simulink model "untitled0"  (R2023a)
settings: Solver=FixedStepAuto  StartTime=0.0  StopTime=3  FixedStep=1e-5  RelTol=1e-3
undefined symbols (not defined in the file): J, Ki, Kiv, Kp, Kpv, KT, La, Ra, Tfi, Tfv, UaN
libraries: spsMosfetLib x4, spsDCMachineLib x1, spsDCVoltageSourceLib x1, simulink x1, spsVoltageMeasurementLib x1, sps_lib x1
settings Model: Creator=luand  LastModifiedBy=luand

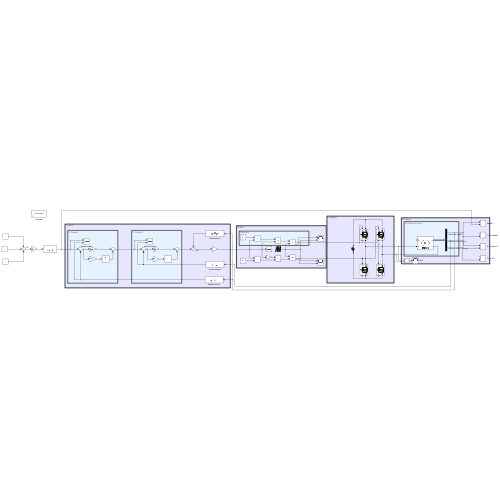
[thumbnail: Simulink's stored preview of the top-level diagram]
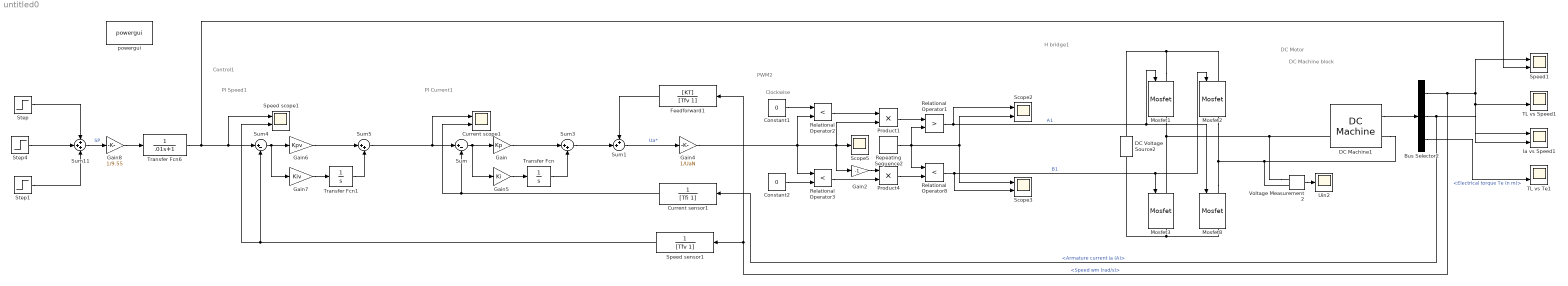
== system untitled0 ==
  note: PI Speed1
  note: PWM2
  note: DC Motor
  note: H bridge1
  note: Control1
  note: DC Machine block
  note: PI Current1
  note: Clockwise
  Bus Selector2 : BusSelector  OutputSignals=Speed wm (rad/s),Armature current ia (A),Electrical torque Te (n m)
  Constant1 : Constant  Value=0
  Constant2 : Constant  Value=0
  Current scope1 : Scope  NumInputPorts=2
  Current sensor1 : TransferFcn  Denominator=[Tfi 1]
  DC Machine1 : spsDCMachineLib/DC Machine  PresetModel=No  MechanicalLoad=Torque TL  FieldType=Permanent magnet  ShowDetailedParameters=on  MeasurementBus=off  RLa=[ Ra La ]  RLf="[ 240  120]"  Laf=1.8  MachineConstant=Torque constant (N.m/A)  Ke=1.8  Kt=KT  J=J  Bm=0  Tf=0  w0=0  Ifinit=1  TsPowergui=0  TsBlock=-1
  DC Voltage Source2 : spsDCVoltageSourceLib/DC Voltage Source  Amplitude=UaN  Measurements=None
  Feedforward1 : TransferFcn  Numerator=[KT]  Denominator=[Tfv 1]
  Gain : Gain  Gain=Kp
  Gain2 : Gain  Gain=-1
  Gain4 : Gain  Gain=1/UaN
  Gain5 : Gain  Gain=Ki
  Gain6 : Gain  Gain=Kpv
  Gain7 : Gain  Gain=Kiv
  Gain8 : Gain  Gain=1/9.55
  Ia vs Speed1 : Scope  NumInputPorts=2
  Mosfet{1..3,8} (4 alike) : spsMosfetLib/Mosfet  Ron=0.1  Lon=0  Rd=0.01  Vfd=0  IC=0  Rs=1e5  Cs=inf  Measurements=on
  Product1 : Product
  Product4 : Product
  Relational Operator1 : RelationalOperator  Operator=>  OutDataTypeStr=boolean  RndMeth=Simplest  InputSameDT=off
  Relational Operator2 : RelationalOperator  Operator=<  OutDataTypeStr=boolean  RndMeth=Simplest  InputSameDT=off
  Relational Operator3 : RelationalOperator  Operator=<  OutDataTypeStr=boolean  RndMeth=Simplest  InputSameDT=off
  Relational Operator8 : RelationalOperator  Operator=<  OutDataTypeStr=boolean  RndMeth=Simplest  InputSameDT=off
  Repeating Sequence2 : simulink/Sources/Repeating Sequence  rep_seq_t=[0 1e-3]  rep_seq_y=[0 1]
  Scope2 : Scope  NumInputPorts=2
  Scope3 : Scope  NumInputPorts=2
  Scope5 : Scope
  Speed scope1 : Scope  NumInputPorts=2
  Speed sensor1 : TransferFcn  Denominator=[Tfv 1]
  Speed1 : Scope  NumInputPorts=2
  Step : Step  Time=0  After=3000  SampleTime=0
  Step1 : Step  Time=2  After=-1500  SampleTime=0
  Step4 : Step  After=-1500  SampleTime=0
  Sum : Sum  Inputs=|+-
  Sum1 : Sum  Inputs=++|
  Sum11 : Sum  Inputs=+++
  Sum3 : Sum  Inputs=|++
  Sum4 : Sum  Inputs=|+-
  Sum5 : Sum  Inputs=|++
  TL vs Speed1 : Scope  NumInputPorts=2
  TL vs Te1 : Scope  NumInputPorts=2
  Transfer Fcn : TransferFcn  Denominator=[1 0]
  Transfer Fcn1 : TransferFcn  Denominator=[1 0]
  Transfer Fcn6 : TransferFcn  Denominator=[.01 1]
  Uin2 : Scope
  Voltage Measurement2 : spsVoltageMeasurementLib/Voltage Measurement  PhasorSimulation=off  OutputType=Complex  PSBequivalent=0
  powergui : sps_lib/powergui  Priority=1  SimulationMode=Continuous  SampleTime=1e-5  frequency=60  Iterations=50  frequencyindice=0  Pbase=100e6  ErrMax=1e-4  UnitsV=kV  UnitsW=MW  buscounter=0  FunctionMessages=off  echomessages=off  EnableUseOfTLC=off  CurrentSourceSwitches=off  DisableSnubberDevices=off  DisableRonSwitches=off  DisableVfSwitches=off  DisplayEquations=off  AutomaticDiscreteSolvers=off  SolverType=Tustin/Backward Euler (TBE)  Interpol=off  ExternalGateDelay=off  methode=off  Ts=100  x0status=blocks  SPID=on  SwTol=0  HookPort=off  NonlinearTolerance=1e-4  nMaxIteration=100  ContinueOnMaxIteration=off  RestoreLinks=warning  ResistiveCurrentMeasurement=off  Frange=[0:2:500]  Ylog=off  Xlog=on  ShowGrid=off  save=off  variable=ZData  structure=0  ZoomFFT=off  StartTime=0.0  cycles=1  DisplayStyle=1  fundamental=60  FreqAxis=off  MaxFrequency=1000  frequencyindicesteady=1  RmsSteady=1  display=off
  wires:
  Constant2/1 -> Relational Operator3/2
  Relational Operator8/1 -> Mosfet2/1, Mosfet3/1, Scope3/2  "B1"
  Product4/1 -> Relational Operator8/2
  Step4/1 -> Sum11/2
  Voltage Measurement2/1 -> Uin2/1
  Sum/1 -> Gain5/1, Gain/1
  Gain7/1 -> Transfer Fcn1/1
  Sum11/1 -> Gain8/1  "SP"
  Bus Selector2/3 -> TL vs Te1/2  "<Electrical torque Te (n m)>"
  Product1/1 -> Relational Operator1/1
  Step1/1 -> Sum11/3
  Step/1 -> Sum11/1
  Gain6/1 -> Sum5/1
  Sum5/1 -> Current scope1/1, Sum/1
  Transfer Fcn/1 -> Sum3/2
  Relational Operator2/1 -> Product1/1
  Transfer Fcn1/1 -> Sum5/2
  Speed sensor1/1 -> Speed scope1/2, Sum4/2
  Constant1/1 -> Relational Operator2/1
  Bus Selector2/1 -> Feedforward1/1, Speed sensor1/1, Ia vs Speed1/2, TL vs Speed1/2, Speed1/1  "<Speed wm (rad/s)>"
  Gain5/1 -> Transfer Fcn/1
  Sum3/1 -> Sum1/2
  Current sensor1/1 -> Current scope1/2, Sum/2
  Transfer Fcn6/1 -> Speed1/2, Speed scope1/1, Sum4/1
  Bus Selector2/2 -> Ia vs Speed1/1, Current sensor1/1  "<Armature current ia (A)>"
  Gain4/1 -> Relational Operator3/1, Product1/2, Gain2/1, Scope5/1, Relational Operator2/2
  Repeating Sequence2/1 -> Relational Operator1/2, Relational Operator8/1, Scope2/2, Scope3/1
  Gain2/1 -> Product4/1
  Relational Operator3/1 -> Product4/2
  Feedforward1/1 -> Sum1/1
  Gain8/1 -> Transfer Fcn6/1
  Gain/1 -> Sum3/1
  Sum1/1 -> Gain4/1  "Ua*"
  Sum4/1 -> Gain7/1, Gain6/1
  Relational Operator1/1 -> Mosfet8/1, Mosfet1/1, Scope2/1  "A1"
  DC Machine1/1 -> Bus Selector2/1
  connections:
  Mosfet8/RConn1 -- Mosfet3/RConn1 -- DC Voltage Source2/LConn1
  Voltage Measurement2/LConn1 -- Mosfet3/LConn1 -- Mosfet1/RConn1 -- DC Machine1/LConn1
  Mosfet1/LConn1 -- Mosfet2/LConn1 -- DC Voltage Source2/RConn1
  Mosfet8/LConn1 -- Voltage Measurement2/LConn2 -- DC Machine1/RConn1 -- Mosfet2/RConn1
